simulink model "HW1_1"  (R2022b)
settings: Solver=VariableStepAuto  StartTime=0.0  StopTime=6  FixedStep=0.0001  MaxStep=0.001  RelTol=1e-3
values from neighbouring files (symbols this model uses):
  Kd = 1000*eye(4)    [HW_par.m]
  Kp = 1000*eye(4)    [HW_par.m]
  q_0 = [0;0;0;0]    [HW_par.m]
  q_dot_0 = [0;0;0;0]    [HW_par.m]
  q_target = [pi/2; pi/3; 0.1; -pi/4]    [HW_par.m]
undefined symbols (not defined in the file or in its folder): a_filt, b_filt
settings Model: Creator=Alberto  LastModifiedBy=emanuelevitetta
settings SolverCC: AlgebraicLoopSolver=TrustRegion
settings DebuggingCC: UnconnectedInputMsg=warning  UnconnectedOutputMsg=warning  UnconnectedLineMsg=warning  SFMachineParentedDataDiag=warning
settings ModelReferenceCC: EnableRefExpFcnMdlSchedulingChecks=on
settings RTWCC: DLArmComputeVersion=19.05

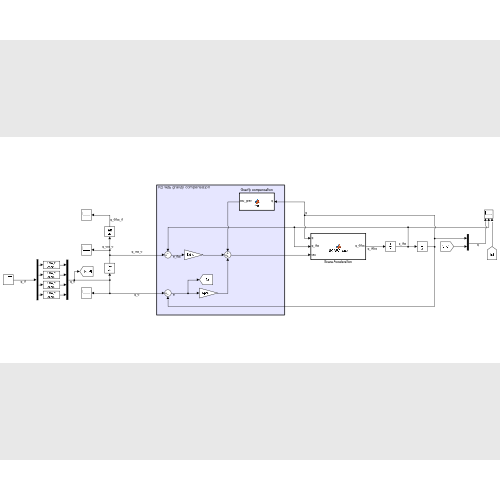
[thumbnail: Simulink's stored preview of the top-level diagram]
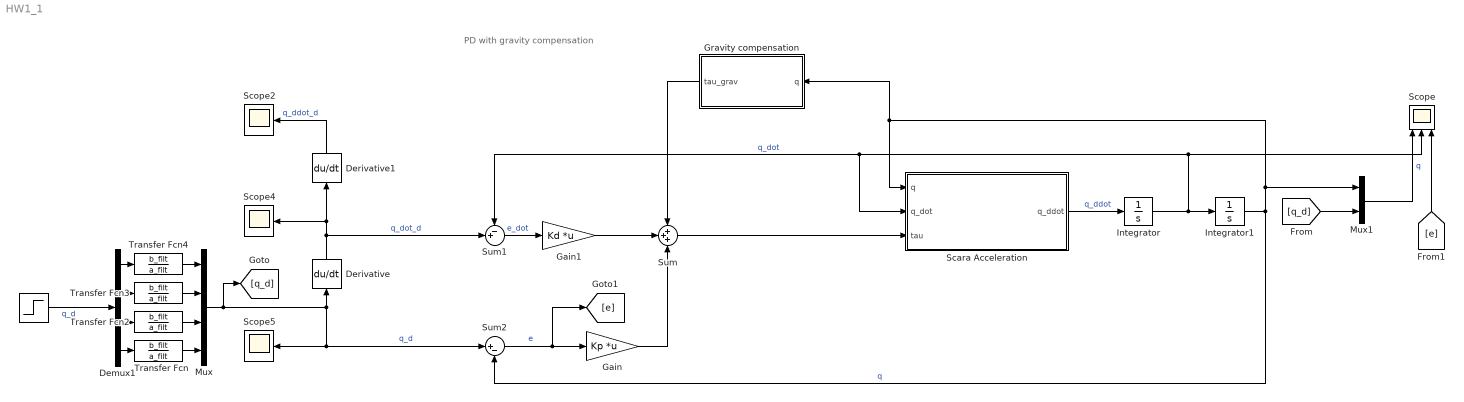
== system HW1_1 ==
  note: PD with gravity compensation
  " " : Step  Before=q_0  After=q_target  SampleTime=0
  Demux1 : Demux
  Derivative : Derivative
  Derivative1 : Derivative
  Gain : Gain  Gain=Kp  Multiplication=Matrix(K*u)
  Gain1 : Gain  Gain=Kd  Multiplication=Matrix(K*u)
  Gravity compensation : MATLAB Function  TreatAsAtomicUnit=on
  Integrator : Integrator  InitialCondition=q_dot_0
  Integrator1 : Integrator  InitialCondition=q_0
  Mux : Mux
  Mux1 : Mux  Inputs=2
  Scara Acceleration : MATLAB Function  TreatAsAtomicUnit=on
  Scope : Scope  NumInputPorts=3
  Scope2 : Scope
  Scope4 : Scope
  Scope5 : Scope
  Sum : Sum  Inputs=+++
  Sum1 : Sum  Inputs=-+|
  Sum2 : Sum  Inputs=|+-
  Transfer Fcn{,2..4} (4 alike) : TransferFcn  Numerator=b_filt  Denominator=a_filt
  wires:
  Demux1/1 -> Transfer Fcn4/1
  Demux1/2 -> Transfer Fcn3/1
  Demux1/3 -> Transfer Fcn2/1
  Demux1/4 -> Transfer Fcn/1
  Transfer Fcn4/1 -> Mux/1
  Transfer Fcn3/1 -> Mux/2
  Transfer Fcn2/1 -> Mux/3
  Transfer Fcn/1 -> Mux/4
  Derivative1/1 -> Scope2/1  "q_ddot_d"
  " "/1 -> Demux1/1  "q_d"
  Integrator1/1 -> Gravity compensation/1(q), Scara Acceleration/1(q), Mux1/1, Sum2/2  "q"
  Gravity compensation/1(tau_grav) -> Sum/1
  Sum/1 -> Scara Acceleration/3(tau)
  Derivative/1 -> Sum1/2, Derivative1/1, Scope4/1  "q_dot_d"
  Mux/1 -> [q_d], Sum2/1, Scope5/1, Derivative/1  "q_d"
  Gain1/1 -> Sum/2
  Sum2/1 -> [e], Gain/1  "e"
  Sum1/1 -> Gain1/1  "e_dot"
  Gain/1 -> Sum/3
  Scara Acceleration/1(q_ddot) -> Integrator/1  "q_ddot"
  Integrator/1 -> Scope/2, Scara Acceleration/2(q_dot), Sum1/1, Integrator1/1  "q_dot"
  Mux1/1 -> Scope/1  "q"
  [e] -> Scope/3
  [q_d] -> Mux1/2

== matlab function HW1_1/Scara Acceleration ==
  data: q input; q_ddot output; q_dot input; tau input
function q_ddot = SCARA_acc(q, q_dot, tau)%#codegen
coder.extrinsic('f_B_mex'); 
coder.extrinsic('f_C_vect_mex'); 
coder.extrinsic('f_g_vect_mex');
B = eye(4);
C_vect = zeros(4,1);
F_g = zeros(4,1);
tau = reshape(tau,4,1);
q_ddot = zeros(4,1);
B = full(f_B_mex('f_B',q));
C_vect = full(f_C_vect_mex('f_C_vect', q, q_dot));
F_g = full(f_g_vect_mex('f_g_vect', q));
q_ddot = (eye(4)/B)*(-C_vect-F_g+tau);

== matlab function HW1_1/Gravity compensation ==
  data: q input; tau_grav output
function tau_grav = fcn(q)%#codegen
coder.extrinsic('f_g_vect_mex');
tau_grav = zeros(4,1);
tau_grav = reshape(full(f_g_vect_mex('f_g_vect', q)),4,1);
